simulink model "continuous_model_linearized"  (R2023b)
settings: Solver=VariableStepAuto  StartTime=0.0  StopTime=t_fin  RelTol=1e-3
InitFcn:
  | model_setup
values from neighbouring files (symbols this model uses):
  a0 = 0.00376903    [model_setup.m]
  a1 = 0.0731193    [model_setup.m]
  a2 = 0.469961    [model_setup.m]
  alpha1 = 0.42    [model_setup.m]
  alpha2 = 0.19    [model_setup.m]
  alpha3 = 1.5    [model_setup.m]
  alpha4 = 0.95    [model_setup.m]
  b0 = 0.0050882    [model_setup.m]
  lin_point = -0.8    [ex2_ex3.m]    (also in ex6.m = lin_points(j); model_setup.m = 0.8)
  u_max = u_maxs(i)    [ex6.m]    (also in ex8.m = 0.5; model_setup.m = 1)
  u_min = 0    [ex6.m]    (also in ex8.m; model_setup.m = -1)
  u_step_time = 10    [model_setup.m]
settings Model: Creator=vistek528  LastModifiedBy=vistek528
settings DataIOCC: ReturnWorkspaceOutputs=off

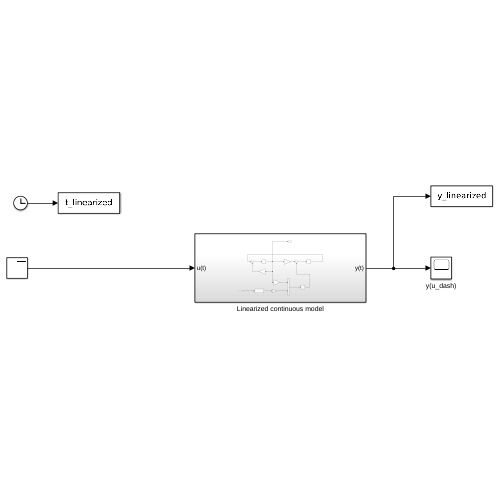
[thumbnail: Simulink's stored preview of the top-level diagram]
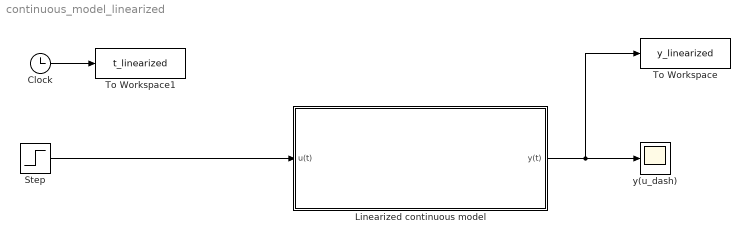
== system continuous_model_linearized ==
  Clock : Clock
  Linearized continuous model : Subsystem
  Step : Step  Time=u_step_time  Before=u_min  After=u_max  SampleTime=0
  To Workspace : ToWorkspace  VariableName=y_linearized  SaveFormat=Timeseries  SampleTime=-1
  To Workspace1 : ToWorkspace  VariableName=t_linearized  SaveFormat=Timeseries  SampleTime=-1
  y(u_dash) : Scope
  wires:
  Clock/1 -> To Workspace1/1
  Step/1 -> Linearized continuous model/1(u(t))
  Linearized continuous model/1(y(t)) -> To Workspace/1, y(u_dash)/1

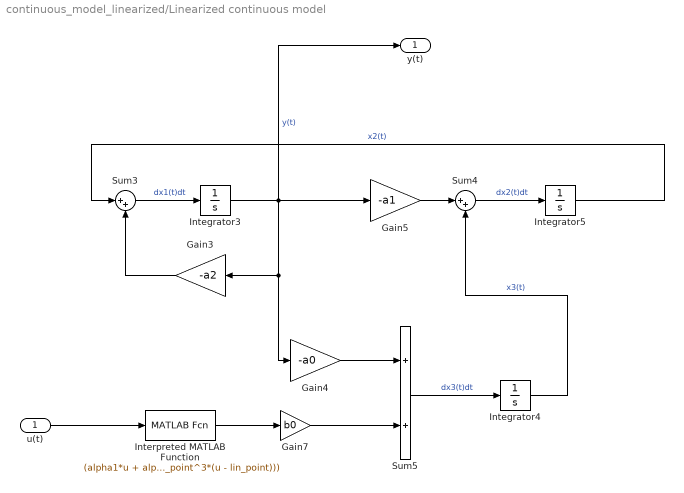
== system continuous_model_linearized/Linearized continuous model ==
  u(t) : Inport
  Gain3 : Gain  Gain=-a2
  Gain4 : Gain  Gain=-a0
  Gain5 : Gain  Gain=-a1
  Gain7 : Gain  Gain=b0
  Integrator3 : Integrator
  Integrator4 : Integrator
  Integrator5 : Integrator
  Interpreted MATLAB Function : MATLABFcn  MATLABFcn=(alpha1*u + alpha2*(2*lin_point*(u - lin_point) + lin_point^2) + alpha3*(lin_point^3 + 3*lin_point^2*(u - lin_point)) + alpha4*(lin_point^4 + 4*lin_point^3*(u - lin_point)))
  Sum3 : Sum  Inputs=|++
  Sum4 : Sum  Inputs=|++
  Sum5 : Sum
  y(t) : Outport
  wires:
  Integrator4/1 -> Sum4/2  "x3(t)"
  Sum3/1 -> Integrator3/1  "dx1(t)dt"
  Gain5/1 -> Sum4/1
  Gain4/1 -> Sum5/1
  Gain7/1 -> Sum5/2
  Integrator3/1 -> y(t)/1, Gain5/1, Gain4/1, Gain3/1  "y(t)"
  Sum4/1 -> Integrator5/1  "dx2(t)dt"
  Sum5/1 -> Integrator4/1  "dx3(t)dt"
  Interpreted MATLAB Function/1 -> Gain7/1
  Integrator5/1 -> Sum3/1  "x2(t)"
  Gain3/1 -> Sum3/2
  u(t)/1 -> Interpreted MATLAB Function/1
